simulink model "System_Twist_Space"  (R2023a)
settings: Solver=VariableStepAuto  StartTime=0.0  StopTime=10  FixedStep=.001  MaxStep=.001  RelTol=1e-6  EnableMultiTasking=on
values from neighbouring files (symbols this model uses):
  Kd = Kd    [SimRun_InvDynamics.m]    (also in SimRun_ThetaSpace.m = [75;75;75;40;1;1]; SimRun_TwistSpace.m = [75;75;75;40;1;1]; project_pt5_controller.m = place(Ad, Bd, cl_poles_disc))
  Ki = Ki * 5    [SimRun_ThetaSpace.m]    (also in SimRun_TwistSpace.m = Ki * 0)
  Kp = Kp * 2    [SimRun_InvDynamics.m]    (also in SimRun_ThetaSpace.m = Kp * 20; SimRun_TwistSpace.m = [500;500;500;300;10;10])
  KpC = [KpRot;KpRot;KpRot;KpDisp;KpDisp;KpDisp]    [SimRun_TwistSpace.m]
undefined symbols (not defined in the file or in its folder): DiscIntNeverNeededParam
(part 1 of 4)
settings Model: Creator=Andrew Petruska  LastModifiedBy=chris
settings SolverCC: AlgebraicLoopSolver=TrustRegion
settings DataIOCC: ReturnWorkspaceOutputs=off
settings OptimizationCC: LifeSpan=inf
settings DebuggingCC: UnconnectedInputMsg=warning  UnconnectedOutputMsg=warning  UnconnectedLineMsg=warning  SFUnexpectedBacktrackingDiag=warning  SFNoUnconditionalDefaultTransitionDiag=warning  ArithmeticOperatorsInVariantConditions=warning
settings ModelReferenceCC: EnableRefExpFcnMdlSchedulingChecks=on
settings SFSimCC: SimUseLocalCustomCode=off  CustomCodeUndefinedFunction=UseInterfaceOnly
settings RTWCC: RTWUseLocalCustomCode=off
settings CodeAppCC: StateflowObjectComments=on
settings GRTTargetCC: TargetLangStandard=C89/C90 (ANSI)
settings ConfigComp: CovMetricSettings=dw  CovSaveCumulativeToWorkspaceVar=on  CovSaveSingleToWorkspaceVar=on  CovExternalEMLEnable=off

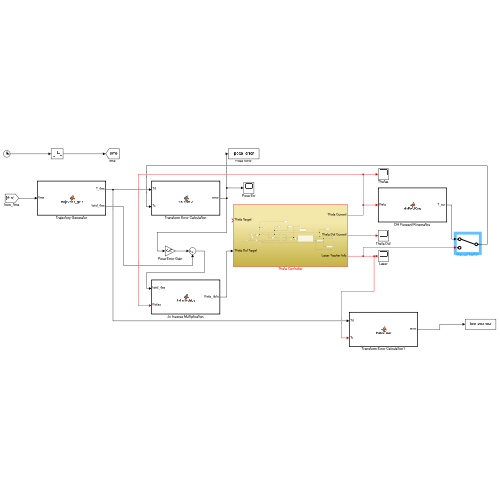
[thumbnail: Simulink's stored preview of the top-level diagram]
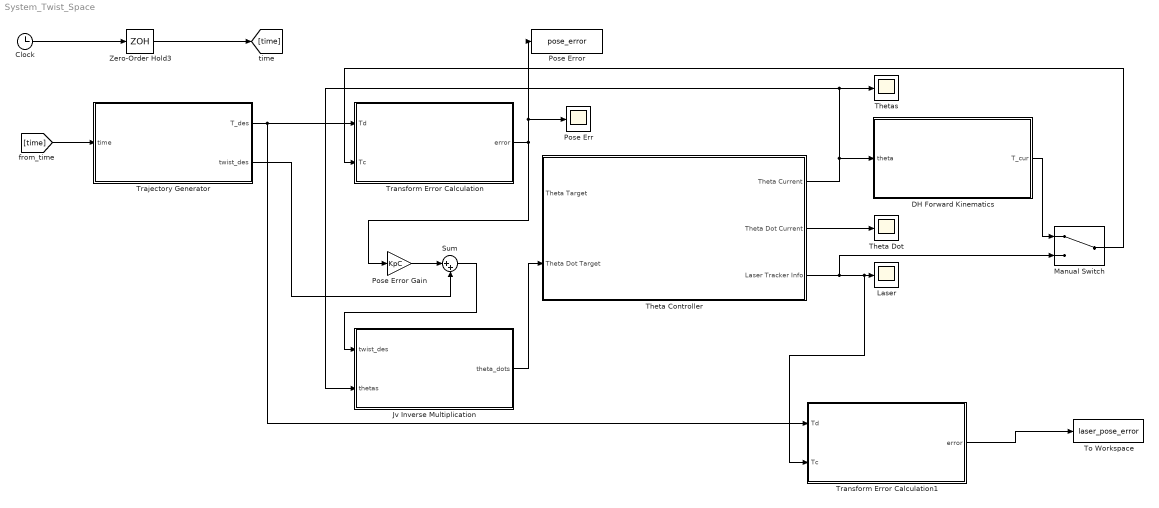
== system System_Twist_Space ==
  Clock : Clock
  DH Forward Kinematics : MATLAB Function  TreatAsAtomicUnit=on
  Jv Inverse Multiplication : MATLAB Function  TreatAsAtomicUnit=on
  Laser : Scope
  Manual Switch : ManualSwitch
  Pose Err : Scope
  Pose Error : ToWorkspace  VariableName=pose_error  SaveFormat=Timeseries  SampleTime=-1
  Pose Error Gain : Gain  Gain=KpC
  Sum : Sum  Inputs=|++
  Theta Controller : Subsystem
  Theta Dot : Scope
  Thetas : Scope
  To Workspace : ToWorkspace  VariableName=laser_pose_error  SaveFormat=Timeseries  SampleTime=-1
  Trajectory Generator : MATLAB Function  TreatAsAtomicUnit=on
  Transform Error Calculation : MATLAB Function  TreatAsAtomicUnit=on
  Transform Error Calculation1 : MATLAB Function  TreatAsAtomicUnit=on
  Zero-Order Hold3 : ZeroOrderHold  SampleTime=0.001
  wires:
  Manual Switch/1 -> Transform Error Calculation/2(Tc)
  Jv Inverse Multiplication/1(theta_dots) -> Theta Controller/2(Theta Dot Target)
  DH Forward Kinematics/1(T_cur) -> Manual Switch/1
  Clock/1 -> Zero-Order Hold3/1
  Theta Controller/1(Theta Current) -> Jv Inverse Multiplication/2(thetas), Thetas/1, DH Forward Kinematics/1(theta)
  Sum/1 -> Jv Inverse Multiplication/1(twist_des)
  Trajectory Generator/2(twist_des) -> Sum/2
  Pose Error Gain/1 -> Sum/1
  Theta Controller/2(Theta Dot Current) -> Theta Dot/1
  Transform Error Calculation/1(error) -> Pose Error/1, Pose Err/1, Pose Error Gain/1
  Trajectory Generator/1(T_des) -> Transform Error Calculation1/1(Td), Transform Error Calculation/1(Td)
  Theta Controller/3(Laser Tracker Info) -> Transform Error Calculation1/2(Tc), Laser/1, Manual Switch/2
  Zero-Order Hold3/1 -> [time]
  [time] -> Trajectory Generator/1(time)
  Transform Error Calculation1/1(error) -> To Workspace/1

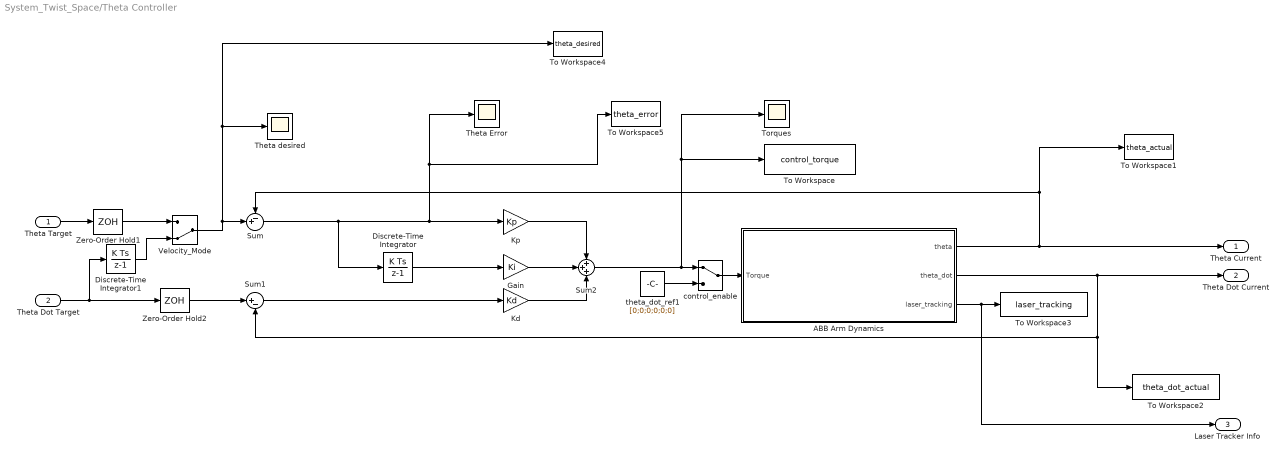
== system System_Twist_Space/Theta Controller ==
  Theta Target : Inport
  Theta Dot Target : Inport  Port=2
  ABB Arm Dynamics : Subsystem
  Discrete-Time Integrator : DiscreteIntegrator  gainval=1  SampleTime=-1  ICPrevOutput=DiscIntNeverNeededParam  ICPrevScaledInput=DiscIntNeverNeededParam
  Discrete-Time Integrator1 : DiscreteIntegrator  gainval=1  SampleTime=-1  ICPrevOutput=DiscIntNeverNeededParam  ICPrevScaledInput=DiscIntNeverNeededParam
  Gain : Gain  Gain=Ki
  Kd : Gain  Gain=Kd
  Kp : Gain  Gain=Kp
  Sum : Sum  Inputs=-+|
  Sum1 : Sum  Inputs=|+-
  Sum2 : Sum  Inputs=+++
  Theta Error : Scope
  Theta desired : Scope
  To Workspace : ToWorkspace  VariableName=control_torque  SaveFormat=Structure With Time  SampleTime=-1
  To Workspace1 : ToWorkspace  VariableName=theta_actual  SaveFormat=Structure With Time  SampleTime=-1
  To Workspace2 : ToWorkspace  VariableName=theta_dot_actual  SaveFormat=Structure With Time  SampleTime=-1
  To Workspace3 : ToWorkspace  VariableName=laser_tracking  SaveFormat=Structure With Time  SampleTime=-1
  To Workspace4 : ToWorkspace  VariableName=theta_desired  SaveFormat=Structure With Time  SampleTime=-1
  To Workspace5 : ToWorkspace  VariableName=theta_error  SaveFormat=Structure With Time  SampleTime=-1
  Torques : Scope
  Velocity_Mode : ManualSwitch  CurrentSetting=0
  Zero-Order Hold1 : ZeroOrderHold  SampleTime=0.001
  Zero-Order Hold2 : ZeroOrderHold  SampleTime=0.001
  control_enable : ManualSwitch
  theta_dot_ref1 : Constant  Value=[0;0;0;0;0;0]
  Theta Current : Outport
  Theta Dot Current : Outport  Port=2
  Laser Tracker Info : Outport  Port=3
  wires:
  control_enable/1 -> ABB Arm Dynamics/1(Torque)
  ABB Arm Dynamics/1(theta) -> Sum/1, To Workspace1/1, Theta Current/1
  Sum/1 -> Discrete-Time Integrator/1, To Workspace5/1, Theta Error/1, Kp/1
  ABB Arm Dynamics/2(theta_dot) -> Sum1/2, To Workspace2/1, Theta Dot Current/1
  Sum2/1 -> To Workspace/1, Torques/1, control_enable/1
  Discrete-Time Integrator/1 -> Gain/1
  theta_dot_ref1/1 -> control_enable/2
  ABB Arm Dynamics/3(laser_tracking) -> Laser Tracker Info/1, To Workspace3/1
  Sum1/1 -> Kd/1
  Kp/1 -> Sum2/1
  Gain/1 -> Sum2/2
  Kd/1 -> Sum2/3
  Theta Target/1 -> Zero-Order Hold1/1
  Theta Dot Target/1 -> Discrete-Time Integrator1/1, Zero-Order Hold2/1
  Zero-Order Hold2/1 -> Sum1/1
  Velocity_Mode/1 -> To Workspace4/1, Theta desired/1, Sum/2
  Zero-Order Hold1/1 -> Velocity_Mode/1
  Discrete-Time Integrator1/1 -> Velocity_Mode/2

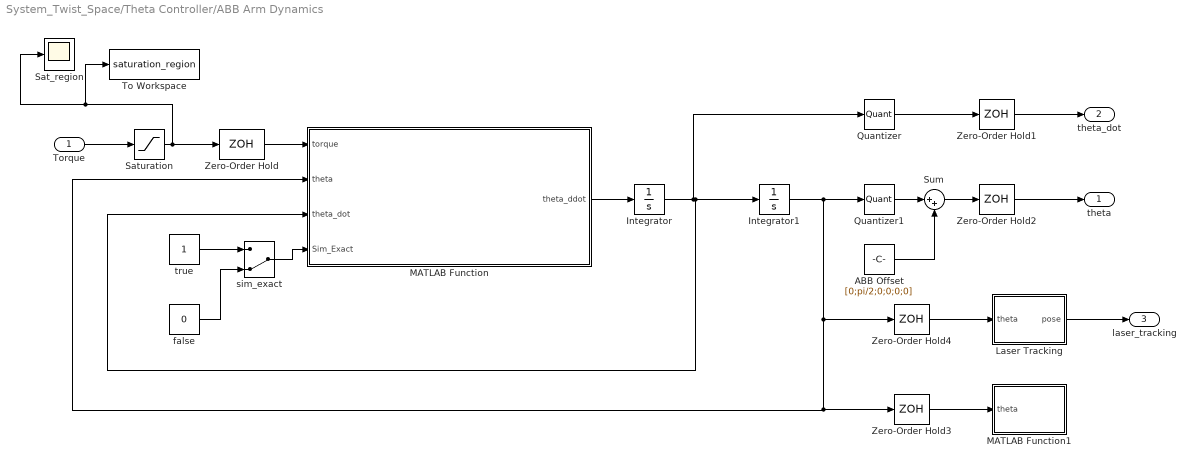
== system System_Twist_Space/Theta Controller/ABB Arm Dynamics ==
  Torque : Inport
  ABB Offset : Constant  Value=[0;pi/2;0;0;0;0]
  Integrator : Integrator  InitialCondition=zeros(6,1)
  Integrator1 : Integrator  InitialCondition=zeros(6,1)
  Laser Tracking : MATLAB Function  TreatAsAtomicUnit=on
  MATLAB Function : MATLAB Function  TreatAsAtomicUnit=on
  MATLAB Function1 : MATLAB Function  TreatAsAtomicUnit=on
  Quantizer : Quantizer  QuantizationInterval=1/2^32
  Quantizer1 : Quantizer  QuantizationInterval=1/2^32
  Sat_region : Scope
  Saturation : Saturate  UpperLimit=350  LowerLimit=-350
  Sum : Sum  Inputs=|++
  To Workspace : ToWorkspace  VariableName=saturation_region  SaveFormat=Timeseries  SampleTime=-1
  Zero-Order Hold{,1..2,4} (4 alike) : ZeroOrderHold  SampleTime=0.001
  Zero-Order Hold3 : ZeroOrderHold  SampleTime=.05
  false : Constant  Value=0
  sim_exact : ManualSwitch  CurrentSetting=0
  true : Constant
  theta : Outport
  theta_dot : Outport  Port=2
  laser_tracking : Outport  Port=3
  wires:
  MATLAB Function/1(theta_ddot) -> Integrator/1
  Integrator/1 -> Quantizer/1, MATLAB Function/3(theta_dot), Integrator1/1
  Zero-Order Hold/1 -> MATLAB Function/1(torque)
  Quantizer/1 -> Zero-Order Hold1/1
  Zero-Order Hold1/1 -> theta_dot/1
  Zero-Order Hold2/1 -> theta/1
  Integrator1/1 -> Quantizer1/1, MATLAB Function/2(theta), Zero-Order Hold3/1, Zero-Order Hold4/1
  Zero-Order Hold3/1 -> MATLAB Function1/1(theta)
  Sum/1 -> Zero-Order Hold2/1
  Quantizer1/1 -> Sum/1
  ABB Offset/1 -> Sum/2
  Laser Tracking/1(pose) -> laser_tracking/1
  Saturation/1 -> Sat_region/1, To Workspace/1, Zero-Order Hold/1
  Zero-Order Hold4/1 -> Laser Tracking/1(theta)
  sim_exact/1 -> MATLAB Function/4(Sim_Exact)
  true/1 -> sim_exact/1
  false/1 -> sim_exact/2
  Torque/1 -> Saturation/1

== matlab function System_Twist_Space/Jv Inverse Multiplication ==
  data: twist_des input; theta_dots output; thetas input
function theta_dots  = JvInvMultipy(twist_des, thetas)
%#codegen
coder.extrinsic('evalin');
coder.extrinsic('min');
coder.extrinsic('length');
coder.extrinsic('velocityJacobian');

persistent linkList;

if isempty(linkList)
    linkList = evalin('base','linkList');
end

% Pre-allocate for Simulink
theta_dots = zeros(6,1);

Jv = velocityJacobian(linkList, thetas);
[U,S,V] = svd(Jv);
S_t = pinv(S,0.002);
Jv_inv = V*S_t*U';
theta_dots = Jv_inv * twist_des;

end

== matlab function System_Twist_Space/Transform Error Calculation1 ==
  data: Td input; error output; Tc input
function error  = transError(Td, Tc)
%#codegen
coder.extrinsic('evalin');
coder.extrinsic('min');
coder.extrinsic('length');
coder.extrinsic('transError');

% Pre-allocate for Simulink
error = zeros(6,1);

error = transError(Td, Tc);

end

== matlab function System_Twist_Space/Trajectory Generator ==
  data: time input; T_des output; twist_des output
function [T_des, twist_des] = trajectory_gen( time )
%#codegen
coder.extrinsic('evalin');
coder.extrinsic('min');
coder.extrinsic('length');
coder.extrinsic('getTwistDesired');

persistent trajectory traj_length index;

if isempty(trajectory) || time == 0
    trajectory = evalin('base','trajectory');
    traj_length = evalin('base','traj_length');
    index = 1;
end

t_point = 0;% pre allocate for simulink
t_point = trajectory(index,1);
if time > t_point
    index = min(traj_length,index+1);
end

% Pre-allocate for Simulink
T_des = zeros(4,4); 
twist_des = zeros(6,1);
[twist_des, T_des] = getTwistDesired(trajectory, time, 0.2);

end

== matlab function System_Twist_Space/Transform Error Calculation ==
  data: Td input; error output; Tc input
function error  = transError(Td, Tc)
%#codegen
coder.extrinsic('evalin');
coder.extrinsic('min');
coder.extrinsic('length');
coder.extrinsic('transError');

% Pre-allocate for Simulink
error = zeros(6,1);

error = transError(Td, Tc);

end

== matlab function System_Twist_Space/DH Forward Kinematics ==
  data: theta input; T_cur output
function T_cur  = dhFwdKine(theta)
%#codegen
coder.extrinsic('evalin');
coder.extrinsic('min');
coder.extrinsic('length');
coder.extrinsic('dhFwdKine');

persistent linkList
if isempty(linkList)
    linkList = evalin('base','linkList');
end

% Pre-allocate for Simulink
T_cur = zeros(4);

T_cur = dhFwdKine(linkList, theta);

end

== matlab function System_Twist_Space/Theta Controller/ABB Arm Dynamics/Laser Tracking ==
  data: theta input; pose output
function pose = laserTracker(theta)
%#codegen
coder.extrinsic('evalin');
persistent Sim_Exact;

if isempty(Sim_Exact)
    Sim_Exact = evalin('base','Sim_Exact');
end


th1 = theta(1);
th2 = theta(2);
th3 = theta(3);
th4 = theta(4);
th5 = theta(5);
th6 = theta(6);


if(Sim_Exact)
    pose = [ sin(th6)*(cos(th4)*sin(th1) + sin(th4)*(cos(th1)*sin(th2)*sin(th3) - cos(th1)*cos(th2)*cos(th3))) + cos(th6)*(cos(th5)*(sin(th1)*sin(th4) - cos(th4)*(cos(th1)*sin(th2)*sin(th3) - cos(th1)*cos(th2)*cos(th3))) - sin(th5)*(cos(th1)*cos(th2)*sin(th3) + cos(th1)*cos(th3)*sin(th2))), cos(th6)*(cos(th4)*sin(th1) + sin(th4)*(cos(th1)*sin(th2)*sin(th3) - cos(th1)*cos(th2)*cos(th3))) - sin(th6)*(cos(th5)*(sin(th1)*sin(th4) - cos(th4)*(cos(th1)*sin(th2)*sin(th3) - cos(th1)*cos(th2)*cos(th3))) - sin(th5)*(cos(th1)*cos(th2)*sin(th3) + cos(th1)*cos(th3)*sin(th2))), - sin(th5)*(sin(th1)*sin(th4) - cos(th4)*(cos(th1)*sin(th2)*sin(th3) - cos(th1)*cos(th2)*cos(th3))) - cos(th5)*(cos(th1)*cos(th2)*sin(th3) + cos(th1)*cos(th3)*sin(th2)), (27*cos(th1)*cos(th2))/100 - (9*sin(th5)*(sin(th1)*sin(th4) - cos(th4)*(cos(th1)*sin(th2)*sin(th3) - cos(th1)*cos(th2)*cos(th3))))/125 - (9*cos(th5)*(cos(th1)*cos(th2)*sin(th3) + cos(th1)*cos(th3)*sin(th2)))/125 - (7*cos(th1)*sin(th2)*sin(th3))/100 + (7*cos(th1)*cos(th2)*cos(th3))/100 - (151*cos(th1)*cos(th2)*sin(th3))/500 - (151*cos(th1)*cos(th3)*sin(th2))/500;
        - sin(th6)*(cos(th1)*cos(th4) - sin(th4)*(sin(th1)*sin(th2)*sin(th3) - cos(th2)*cos(th3)*sin(th1))) - cos(th6)*(cos(th5)*(cos(th1)*sin(th4) + cos(th4)*(sin(th1)*sin(th2)*sin(th3) - cos(th2)*cos(th3)*sin(th1))) + sin(th5)*(cos(th2)*sin(th1)*sin(th3) + cos(th3)*sin(th1)*sin(th2))), sin(th6)*(cos(th5)*(cos(th1)*sin(th4) + cos(th4)*(sin(th1)*sin(th2)*sin(th3) - cos(th2)*cos(th3)*sin(th1))) + sin(th5)*(cos(th2)*sin(th1)*sin(th3) + cos(th3)*sin(th1)*sin(th2))) - cos(th6)*(cos(th1)*cos(th4) - sin(th4)*(sin(th1)*sin(th2)*sin(th3) - cos(th2)*cos(th3)*sin(th1))), sin(th5)*(cos(th1)*sin(th4) + cos(th4)*(sin(th1)*sin(th2)*sin(th3) - cos(th2)*cos(th3)*sin(th1))) - cos(th5)*(cos(th2)*sin(th1)*sin(th3) + cos(th3)*sin(th1)*sin(th2)), (27*cos(th2)*sin(th1))/100 + (9*sin(th5)*(cos(th1)*sin(th4) + cos(th4)*(sin(th1)*sin(th2)*sin(th3) - cos(th2)*cos(th3)*sin(th1))))/125 - (9*cos(th5)*(cos(th2)*sin(th1)*sin(th3) + cos(th3)*sin(th1)*sin(th2)))/125 - (151*cos(th2)*sin(th1)*sin(th3))/500 - (151*cos(th3)*sin(th1)*sin(th2))/500 - (7*sin(th1)*sin(th2)*sin(th3))/100 + (7*cos(th2)*cos(th3)*sin(th1))/100;
        sin(th4)*sin(th6)*(cos(th2)*sin(th3) + cos(th3)*sin(th2)) - cos(th6)*(sin(th5)*(cos(th2)*cos(th3) - sin(th2)*sin(th3)) + cos(th4)*cos(th5)*(cos(th2)*sin(th3) + cos(th3)*sin(th2))), sin(th6)*(sin(th5)*(cos(th2)*cos(th3) - sin(th2)*sin(th3)) + cos(th4)*cos(th5)*(cos(th2)*sin(th3) + cos(th3)*sin(th2))) + cos(th6)*sin(th4)*(cos(th2)*sin(th3) + cos(th3)*sin(th2)), cos(th4)*sin(th5)*(cos(th2)*sin(th3) + cos(th3)*sin(th2)) - cos(th5)*(cos(th2)*cos(th3) - sin(th2)*sin(th3)), (151*sin(th2)*sin(th3))/500 - (151*cos(th2)*cos(th3))/500 - (7*cos(th2)*sin(th3))/100 - (7*cos(th3)*sin(th2))/100 - (27*sin(th2))/100 - (9*cos(th5)*(cos(th2)*cos(th3) - sin(th2)*sin(th3)))/125 + (9*cos(th4)*sin(th5)*(cos(th2)*sin(th3) + cos(th3)*sin(th2)))/125 + 29/100;
        0, 0, 0, 1];
else
    
    pose = [ sin(th6)*(cos(th4)*sin(th1) + sin(th4)*(cos(th1)*sin(th2)*sin(th3) - cos(th1)*cos(th2)*cos(th3))) + cos(th6)*(cos(th5)*(sin(th1)*sin(th4) - cos(th4)*(cos(th1)*sin(th2)*sin(th3) - cos(th1)*cos(th2)*cos(th3))) - sin(th5)*(cos(th1)*cos(th2)*sin(th3) + cos(th1)*cos(th3)*sin(th2))), cos(th6)*(cos(th4)*sin(th1) + sin(th4)*(cos(th1)*sin(th2)*sin(th3) - cos(th1)*cos(th2)*cos(th3))) - sin(th6)*(cos(th5)*(sin(th1)*sin(th4) - cos(th4)*(cos(th1)*sin(th2)*sin(th3) - cos(th1)*cos(th2)*cos(th3))) - sin(th5)*(cos(th1)*cos(th2)*sin(th3) + cos(th1)*cos(th3)*sin(th2))), - sin(th5)*(sin(th1)*sin(th4) - cos(th4)*(cos(th1)*sin(th2)*sin(th3) - cos(th1)*cos(th2)*cos(th3))) - cos(th5)*(cos(th1)*cos(th2)*sin(th3) + cos(th1)*cos(th3)*sin(th2)), (151838081588107*cos(th1)*cos(th2))/562949953421312 - (123928564092639*sin(th1))/72057594037927936 - (7184037743251309*cos(th1))/36893488147419103232 - (7330531551818703*cos(th4)*sin(th1))/36893488147419103232 - (5489399374888815*sin(th1)*sin(th4))/9223372036854775808 + (970893499285375*cos(th5)*(sin(th1)*sin(th4) - cos(th4)*(cos(th1)*sin(th2)*sin(th3) - cos(th1)*cos(th2)*cos(th3))))/9223372036854775808 - (5192391675427195*sin(th5)*(sin(th1)*sin(th4) - cos(th4)*(cos(th1)*sin(th2)*sin(th3) - cos(th1)*cos(th2)*cos(th3))))/72057594037927936 + (1663072680156839*sin(th6)*(cos(th4)*sin(th1) + sin(th4)*(cos(th1)*sin(th2)*sin(th3) - cos(th1)*cos(th2)*cos(th3))))/2305843009213693952 + (1663072680156839*cos(th6)*(cos(th5)*(sin(th1)*sin(th4) - cos(th4)*(cos(th1)*sin(th2)*sin(th3) - cos(th1)*cos(th2)*cos(th3))) - sin(th5)*(cos(th1)*cos(th2)*sin(th3) + cos(th1)*cos(th3)*sin(th2))))/2305843009213693952 + (5489399374888815*cos(th4)*(cos(th1)*sin(th2)*sin(th3) - cos(th1)*cos(th2)*cos(th3)))/9223372036854775808 - (5192391675427195*cos(th5)*(cos(th1)*cos(th2)*sin(th3) + cos(th1)*cos(th3)*sin(th2)))/72057594037927936 - (7330531551818703*sin(th4)*(cos(th1)*sin(th2)*sin(th3) - cos(th1)*cos(th2)*cos(th3)))/36893488147419103232 - (970893499285375*sin(th5)*(cos(th1)*cos(th2)*sin(th3) + cos(th1)*cos(th3)*sin(th2)))/9223372036854775808 - (1259578569946919*cos(th1)*sin(th2)*sin(th3))/18014398509481984 + (1259578569946919*cos(th1)*cos(th2)*cos(th3))/18014398509481984 - (5430591396830085*cos(th1)*cos(th2)*sin(th3))/18014398509481984 - (5430591396830085*cos(th1)*cos(th3)*sin(th2))/18014398509481984;
        - sin(th6)*(cos(th1)*cos(th4) - sin(th4)*(sin(th1)*sin(th2)*sin(th3) - cos(th2)*cos(th3)*sin(th1))) - cos(th6)*(cos(th5)*(cos(th1)*sin(th4) + cos(th4)*(sin(th1)*sin(th2)*sin(th3) - cos(th2)*cos(th3)*sin(th1))) + sin(th5)*(cos(th2)*sin(th1)*sin(th3) + cos(th3)*sin(th1)*sin(th2))), sin(th6)*(cos(th5)*(cos(th1)*sin(th4) + cos(th4)*(sin(th1)*sin(th2)*sin(th3) - cos(th2)*cos(th3)*sin(th1))) + sin(th5)*(cos(th2)*sin(th1)*sin(th3) + cos(th3)*sin(th1)*sin(th2))) - cos(th6)*(cos(th1)*cos(th4) - sin(th4)*(sin(th1)*sin(th2)*sin(th3) - cos(th2)*cos(th3)*sin(th1))), sin(th5)*(cos(th1)*sin(th4) + cos(th4)*(sin(th1)*sin(th2)*sin(th3) - cos(th2)*cos(th3)*sin(th1))) - cos(th5)*(cos(th2)*sin(th1)*sin(th3) + cos(th3)*sin(th1)*sin(th2)), (123928564092639*cos(th1))/72057594037927936 - (7184037743251309*sin(th1))/36893488147419103232 + (7330531551818703*cos(th1)*cos(th4))/36893488147419103232 + (151838081588107*cos(th2)*sin(th1))/562949953421312 + (5489399374888815*cos(th1)*sin(th4))/9223372036854775808 - (970893499285375*cos(th5)*(cos(th1)*sin(th4) + cos(th4)*(sin(th1)*sin(th2)*sin(th3) - cos(th2)*cos(th3)*sin(th1))))/9223372036854775808 + (5192391675427195*sin(th5)*(cos(th1)*sin(th4) + cos(th4)*(sin(th1)*sin(th2)*sin(th3) - cos(th2)*cos(th3)*sin(th1))))/72057594037927936 - (1663072680156839*sin(th6)*(cos(th1)*cos(th4) - sin(th4)*(sin(th1)*sin(th2)*sin(th3) - cos(th2)*cos(th3)*sin(th1))))/2305843009213693952 + (5489399374888815*cos(th4)*(sin(th1)*sin(th2)*sin(th3) - cos(th2)*cos(th3)*sin(th1)))/9223372036854775808 - (5192391675427195*cos(th5)*(cos(th2)*sin(th1)*sin(th3) + cos(th3)*sin(th1)*sin(th2)))/72057594037927936 - (1663072680156839*cos(th6)*(cos(th5)*(cos(th1)*sin(th4) + cos(th4)*(sin(th1)*sin(th2)*sin(th3) - cos(th2)*cos(th3)*sin(th1))) + sin(th5)*(cos(th2)*sin(th1)*sin(th3) + cos(th3)*sin(th1)*sin(th2))))/2305843009213693952 - (7330531551818703*sin(th4)*(sin(th1)*sin(th2)*sin(th3) - cos(th2)*cos(th3)*sin(th1)))/36893488147419103232 - (970893499285375*sin(th5)*(cos(th2)*sin(th1)*sin(th3) + cos(th3)*sin(th1)*sin(th2)))/9223372036854775808 - (5430591396830085*cos(th2)*sin(th1)*sin(th3))/18014398509481984 - (5430591396830085*cos(th3)*sin(th1)*sin(th2))/18014398509481984 - (1259578569946919*sin(th1)*sin(th2)*sin(th3))/18014398509481984 + (1259578569946919*cos(th2)*cos(th3)*sin(th1))/18014398509481984;
        sin(th4)*sin(th6)*(cos(th2)*sin(th3) + cos(th3)*sin(th2)) - cos(th6)*(sin(th5)*(cos(th2)*cos(th3) - sin(th2)*sin(th3)) + cos(th4)*cos(th5)*(cos(th2)*sin(th3) + cos(th3)*sin(th2))), sin(th6)*(sin(th5)*(cos(th2)*cos(th3) - sin(th2)*sin(th3)) + cos(th4)*cos(th5)*(cos(th2)*sin(th3) + cos(th3)*sin(th2))) + cos(th6)*sin(th4)*(cos(th2)*sin(th3) + cos(th3)*sin(th2)), cos(th4)*sin(th5)*(cos(th2)*sin(th3) + cos(th3)*sin(th2)) - cos(th5)*(cos(th2)*cos(th3) - sin(th2)*sin(th3)), (5430591396830085*sin(th2)*sin(th3))/18014398509481984 - (5430591396830085*cos(th2)*cos(th3))/18014398509481984 - (1259578569946919*cos(th2)*sin(th3))/18014398509481984 - (1259578569946919*cos(th3)*sin(th2))/18014398509481984 - (1663072680156839*cos(th6)*(sin(th5)*(cos(th2)*cos(th3) - sin(th2)*sin(th3)) + cos(th4)*cos(th5)*(cos(th2)*sin(th3) + cos(th3)*sin(th2))))/2305843009213693952 - (151838081588107*sin(th2))/562949953421312 + (5489399374888815*cos(th4)*(cos(th2)*sin(th3) + cos(th3)*sin(th2)))/9223372036854775808 - (5192391675427195*cos(th5)*(cos(th2)*cos(th3) - sin(th2)*sin(th3)))/72057594037927936 - (7330531551818703*sin(th4)*(cos(th2)*sin(th3) + cos(th3)*sin(th2)))/36893488147419103232 - (970893499285375*sin(th5)*(cos(th2)*cos(th3) - sin(th2)*sin(th3)))/9223372036854775808 - (970893499285375*cos(th4)*cos(th5)*(cos(th2)*sin(th3) + cos(th3)*sin(th2)))/9223372036854775808 + (5192391675427195*cos(th4)*sin(th5)*(cos(th2)*sin(th3) + cos(th3)*sin(th2)))/72057594037927936 + (1663072680156839*sin(th4)*sin(th6)*(cos(th2)*sin(th3) + cos(th3)*sin(th2)))/2305843009213693952 + 325695105792877/1125899906842624;
        0, 0, 0, 1];
end
